simulink model "ModeAdjust"  (R2018b)
settings: Solver=FixedStepDiscrete  StartTime=0.0  StopTime=inf  FixedStep=0.01  RelTol=1e-3
undefined symbols (not defined in the file or in its folder): IfKeSMSbSeatMovBkRclnEnable_Val, IfKeSMSbSeatMovFrwdBkwdEnable_Val, IfKeSMSbSeatMovFtrstEnable_Val, IfKeSMSbSeatMovHdrstFrwdBkwdEnable_Val, IfKeSMSbSeatMovHdUpwdDnwdEnable_Val, IfKeSMSbSeatMovLgrstEnable_Val, IfKeSMSbSeatMovLtwdRtwdEnable_Val, IfVeSMSeStNumConfig, KeSMSbArmscreenMovEnable_Val, KeSMSbSeatMovLgrstExpdEnable_Val, KeSMSuFirstRwStBackPosDelta_Val, KeSMSuFirstRwStBackPosTolr_Val, KeSMSuFirstRwStCushFrntPosDelta_Val, KeSMSuFirstRwStCushFrntPosTolr_Val, KeSMSuFirstRwStCushRePosDelta_Val, KeSMSuFirstRwStCushRePosTolr_Val, KeSMSuFirstRwStFootrestPosDelta_Val, KeSMSuFirstRwStFootrestPosTolr_Val, KeSMSuFirstRwStFwdBkwdPosDelta_Val, KeSMSuFirstRwStFwdBkwdPosTolr_Val, KeSMSuMdMotFinshdTm_Val, KeSMSuMdRetryTm1_Val, KeSMSuModeReqDurgTm_Val, KeSMSuSecRwStArmTochPosDelta_Val, KeSMSuSecRwStArmTochPosTolr_Val, KeSMSuSecRwStBackPosDelta_Val, KeSMSuSecRwStBackPosTolr_Val, KeSMSuSecRwStFtrstUpwdDnwdPosDelta_Val, KeSMSuSecRwStFtrstUpwdDnwdPosTolr_Val, KeSMSuSecRwStFwdBkwdPosDelta_Val, KeSMSuSecRwStFwdBkwdPosTolr_Val, KeSMSuSecRwStHeadrestFwdBkwdPosDelta_Val, KeSMSuSecRwStHeadrestFwdBkwdPosTolr_Val, KeSMSuSecRwStHeadrestUpwdDwnwdPosDelta_Val, KeSMSuSecRwStHeadrestUpwdDwnwdPosTolr_Val, KeSMSuSecRwStLegrestInOutPosDelta_Val, KeSMSuSecRwStLegrestInOutPosTolr_Val, KeSMSuSecRwStLegrestUpwdDwnwdPosDelta_Val, KeSMSuSecRwStLegrestUpwdDwnwdPosTolr_Val, KeSMSuSecRwStLwdRwdPosDelta_Val, KeSMSuSecRwStLwdRwdPosTolr_Val, KeSMSuSecRwStVIPFtrstRefAngle_Val, KeSMSuThirdRwStFwdBkwdPosDelta_Val, KeSMSuThirdRwStFwdBkwdPosTolr_Val, KeSMSuThrdRwCushFoldPosDelta_Val, KeSMSuThrdRwCushFoldPosTolr_Val, KeSMSuThrdRwStBackPosDelta_Val, KeSMSuThrdRwStBackPosTolr_Val, KeSMSw4SLegrstCloseMdSecRwLtStFtrstUpwdDnwdPos_Val, KeSMSw4SLegrstCloseMdSecRwLtStFtrstUpwdDnwdPosMax_Val, KeSMSw4SLegrstCloseMdSecRwLtStFtrstUpwdDnwdPosMin_Val, KeSMSw4SLegrstCloseMdSecRwLtStLgrstOtwdInwdPos_Val, KeSMSw4SLegrstCloseMdSecRwLtStLgrstOtwdInwdPosMax_Val, KeSMSw4SLegrstCloseMdSecRwLtStLgrstOtwdInwdPosMin_Val, KeSMSw4SLegrstCloseMdSecRwLtStLgrstUpwdDnwdPos_Val, KeSMSw4SLegrstCloseMdSecRwLtStLgrstUpwdDnwdPosMax_Val, KeSMSw4SLegrstCloseMdSecRwLtStLgrstUpwdDnwdPosMin_Val, KeSMSw4SLegrstCloseMdSecRwRtStFtrstUpwdDnwdPos_Val, KeSMSw4SLegrstCloseMdSecRwRtStFtrstUpwdDnwdPosMax_Val, KeSMSw4SLegrstCloseMdSecRwRtStFtrstUpwdDnwdPosMin_Val ... (+1138)
libraries: Lib x401
(part 16 of 35)

== system ModeAdjust/ModeAdjustRunnable_sys/ModeAdjust/FAMLYR/R3Lt ==
  note: %1锁，2未锁
  Mode_Trig : Inport
  Step1En : Inport  Port=2
  ThdRwRtStPoss : Inport  Port=3
  ThdRwRtStPossV : Inport  Port=4
  ModeStCalib_3R : Inport  Port=5
  StConfig : Inport  Port=6
  SecRwRtStChldLkRsp_L : Inport  Port=7
  SecRwRtStChldLkRsp_R : Inport  Port=8
  Bus Creator : BusCreator  Inputs=3  OutDataTypeStr=Bus: ThdRwLfSeatPos
  Bus Selector : BusSelector  OutputSignals=IfVeSMSuThdRwLtStBkReclnUpwdDnwdPos_Val_read,IfVeSMSuThdRwLtStCshnFldUpwdDnwdPos_Val_read,IfVeSMSuThdRwLtStFrwdBkwdPos_Val_read
  Bus Selector1 : BusSelector  OutputSignals=IfVeSMSuThdRwLtStBkReclnUpwdDnwdPosV_Val_read,IfVeSMSuThdRwLtStCshnFldUpwdDnwdPosV_Val_read,IfVeSMSuThdRwLtStFrwdBkwdPosV_Val_read
  Bus Selector2 : BusSelector  OutputSignals=BkReclnUpwdDnwdPos,BkReclnUpwdDnwdPosMax,BkReclnUpwdDnwdPosMin,CshnFldUpwdDnwdPos,CshnFldUpwdDnwdPosMax,CshnFldUpwdDnwdPosMin,FrwdBkwdPos,FrwdBkwdPosMax,FrwdBkwdPosMin
  Bus Selector3 : BusSelector  OutputSignals=FamlyRThdRwLtSt
  Bus Selector4 : BusSelector  OutputSignals=BkReclnUpwdDnwdMovConfig,CshnFldUpwdDnwdMovConfig,FrwdBkwdMovConfig
  Constant : Constant  Value=2  OutDataTypeStr=uint8
  Constant1 : Constant  Value=0  OutDataTypeStr=uint8
  Logical Operator10 : Logic  Operator=OR  AllPortsSameDT=off  OutDataTypeStr=boolean
  Logical Operator6 : Logic  Operator=OR  AllPortsSameDT=off  OutDataTypeStr=boolean
  PA_KeSMSuMdMotFinshdTm_Val : Constant  Value=KeSMSuMdMotFinshdTm_Val
  PA_KeSMSuMdRetryTm1_Val : Constant  Value=KeSMSuMdRetryTm1_Val
  PA_KeSMSuModeReqDurgTm_Val : Constant  Value=KeSMSuModeReqDurgTm_Val
  PA_KeSMSuThirdRwStFwdBkwdPosDelta_Val : Constant  Value=KeSMSuThirdRwStFwdBkwdPosDelta_Val
  PA_KeSMSuThrdRwCushFoldPosDelta_Val : Constant  Value=KeSMSuThrdRwCushFoldPosDelta_Val
  PA_KeSMSuThrdRwStBackPosDelta_Val : Constant  Value=KeSMSuThrdRwStBackPosDelta_Val
  PA_KeSMSwDltTrgtPos_Val{1,6..7,18} (4 alike) : Constant  Value=KeSMSwPosInvalidVal_Val
  PA_KeSMSwDltTrgtPos_Val10 : Constant  OutDataTypeStr=boolean
  PA_KeSMSwDltTrgtPos_Val13 : Constant  Value=SeatChldLkSt.ChldLkSt_Unlock
  PA_KeSMSwDltTrgtPos_Val2 : Constant  Value=0  OutDataTypeStr=boolean
  PA_KeSMSwDltTrgtPos_Val3 : Constant  Value=0  OutDataTypeStr=boolean
  PA_KeSMSwDltTrgtPos_Val4 : Constant  Value=SeatChldLkSt.ChldLkSt_Unlock
  R3Rt_FrwdBkwd_Step2 : Lib/CommonUsed  SystemSampleTime=-1
  Relational Operator : RelationalOperator  Operator=~=  OutDataTypeStr=boolean  RndMeth=Simplest
  Relational Operator1 : RelationalOperator  Operator=~=  OutDataTypeStr=boolean  RndMeth=Simplest
  Relational Operator2 : RelationalOperator  Operator=~=  OutDataTypeStr=boolean  RndMeth=Simplest
  Switch : Switch  Criteria=u2 ~= 0
  Unit Delay : UnitDelay  SampleTime=-1
  R3Rt_Step1_ini : Outport
  R3Lt__Step1done : Outport  Port=2
  IfVeSMSbThdRwLtStRclCmdSrv_Val_writeRaw : Outport  Port=3
  R3Lt_TrgtPoss : Outport  Port=4  VectorParamsAs1DForOutWhenUnconnected=on
  R3Lt_SpdCtrl : Outport  Port=5  VectorParamsAs1DForOutWhenUnconnected=on
  wires:
  Bus Selector2/8 -> [K_FrwdBkwdPosMax]  "<FrwdBkwdPosMax>"
  Bus Selector2/1 -> [K_BkReclnUpwdDnwdPos]  "<BkReclnUpwdDnwdPos>"
  Bus Selector2/2 -> [K_BkReclnUpwdDnwdPosMax]  "<BkReclnUpwdDnwdPosMax>"
  Bus Selector2/9 -> [K_FrwdBkwdPosMin]  "<FrwdBkwdPosMin>"
  Bus Selector3/1 -> Bus Selector2/1  "<FamlyRThdRwLtSt>"
  Bus Selector2/3 -> [K_BkReclnUpwdDnwdPosMin]  "<BkReclnUpwdDnwdPosMin>"
  ModeStCalib_3R/1 -> Bus Selector3/1
  Bus Selector2/5 -> [K_CshnFldUpwdDnwdPosMax]  "<CshnFldUpwdDnwdPosMax>"
  Bus Selector2/7 -> [K_FrwdBkwdPos]  "<FrwdBkwdPos>"
  Bus Selector2/4 -> [K_CshnFldUpwdDnwdPos]  "<CshnFldUpwdDnwdPos>"
  Bus Selector2/6 -> [K_CshnFldUpwdDnwdPosMin]  "<CshnFldUpwdDnwdPosMin>"
  [KeSMSuMdMotFinshdTm_Val] -> R3Rt_FrwdBkwd_Step2/12
  PA_KeSMSuModeReqDurgTm_Val/1 -> [Tick]
  PA_KeSMSuMdMotFinshdTm_Val/1 -> [KeSMSuMdMotFinshdTm_Val]
  PA_KeSMSuThrdRwStBackPosDelta_Val/1 -> [KeSMSuThrdRwStBackPosDelta_Val]
  PA_KeSMSuThirdRwStFwdBkwdPosDelta_Val/1 -> [KeSMSuThirdRwStFwdBkwdPosDelta_Val]
  PA_KeSMSuThrdRwCushFoldPosDelta_Val/1 -> [KeSMSuThrdRwCushFoldPosDelta_Val]
  Logical Operator6/1 -> R3Lt__Step1done/1
  Unit Delay/1 -> Logical Operator6/2
  Step1En/1 -> R3Rt_FrwdBkwd_Step2/2
  [Step1_2_done] -> Unit Delay/1
  [R3Rt_Step1_2_ini] -> Logical Operator6/1, R3Rt_Step1_ini/1
  Mode_Trig/1 -> [Trig]
  [ThdRwRtStFrwdBkwdPos] -> R3Rt_FrwdBkwd_Step2/3
  [K_FrwdBkwdPosMax] -> R3Rt_FrwdBkwd_Step2/5
  [KeSMSuThirdRwStFwdBkwdPosDelta_Val] -> R3Rt_FrwdBkwd_Step2/7
  [K_FrwdBkwdPosMin] -> R3Rt_FrwdBkwd_Step2/4
  R3Rt_FrwdBkwd_Step2/1 -> [R3Rt_Step1_2_ini]
  R3Rt_FrwdBkwd_Step2/2 -> [Step2ArrivedTarPos]
  [Trig] -> R3Rt_FrwdBkwd_Step2/1
  [K_FrwdBkwdPos] -> R3Rt_FrwdBkwd_Step2/6
  [ThdRwRtStFrwdBkwdPosV] -> R3Rt_FrwdBkwd_Step2/8
  PA_KeSMSwDltTrgtPos_Val2/1 -> R3Rt_FrwdBkwd_Step2/9
  PA_KeSMSwDltTrgtPos_Val6/1 -> R3Rt_FrwdBkwd_Step2/10
  [Tick] -> R3Rt_FrwdBkwd_Step2/11
  R3Rt_FrwdBkwd_Step2/3 -> [R3Rt_FrwdBkwd_TarPos]
  R3Rt_FrwdBkwd_Step2/4 -> [Step1_2_done]
  Bus Selector1/1 -> [ThdRwRtStBkReclnUpwdDnwdPosV]  "<IfVeSMSuThdRwLtStBkReclnUpwdDnwdPosV_Val_read>"
  Bus Selector/3 -> [ThdRwRtStFrwdBkwdPos]  "<IfVeSMSuThdRwLtStFrwdBkwdPos_Val_read>"
  ThdRwRtStPossV/1 -> Bus Selector1/1
  ThdRwRtStPoss/1 -> Bus Selector/1
  Bus Selector/2 -> [ThdRwRtStCshnFldUpwdDnwdPos]  "<IfVeSMSuThdRwLtStCshnFldUpwdDnwdPos_Val_read>"
  Bus Selector/1 -> [ThdRwRtStBkReclnUpwdDnwdPos]  "<IfVeSMSuThdRwLtStBkReclnUpwdDnwdPos_Val_read>"
  Bus Selector1/2 -> [ThdRwRtStCshnFldUpwdDnwdPosV]  "<IfVeSMSuThdRwLtStCshnFldUpwdDnwdPosV_Val_read>"
  Bus Selector1/3 -> [ThdRwRtStFrwdBkwdPosV]  "<IfVeSMSuThdRwLtStFrwdBkwdPosV_Val_read>"
  PA_KeSMSwDltTrgtPos_Val1/1 -> Bus Creator/2  "ThdRwLtStCshnFldUpwdDnwdTrgtPos"
  PA_KeSMSwDltTrgtPos_Val7/1 -> Bus Creator/1  "ThdRwLtStBkReclnUpwdDnwdTrgtPos"
  [R3Rt_FrwdBkwd_TarPos] -> Bus Creator/3  "ThdRwLtStFrwdBkwdTrgtPos"
  Bus Creator/1 -> R3Lt_TrgtPoss/1
  Bus Selector4/1 -> [BkReclnUpwdDnwdMovConfig]  "<BkReclnUpwdDnwdMovConfig>"
  StConfig/1 -> Bus Selector4/1
  Bus Selector4/2 -> [CshnFldUpwdDnwdMovConfig]  "<CshnFldUpwdDnwdMovConfig>"
  Bus Selector4/3 -> [FrwdBkwdMovConfig]  "<FrwdBkwdMovConfig>"
  [FrwdBkwdMovConfig] -> R3Rt_FrwdBkwd_Step2/14
  PA_KeSMSwDltTrgtPos_Val10/1 -> IfVeSMSbThdRwLtStRclCmdSrv_Val_writeRaw/1
  PA_KeSMSwDltTrgtPos_Val3/1 -> R3Rt_FrwdBkwd_Step2/13
  PA_KeSMSwDltTrgtPos_Val13/1 -> Relational Operator1/2
  SecRwRtStChldLkRsp_R/1 -> Relational Operator1/1
  Relational Operator1/1 -> Logical Operator10/2
  SecRwRtStChldLkRsp_L/1 -> Relational Operator/1
  Relational Operator/1 -> Logical Operator10/1
  Logical Operator10/1 -> [ChildLocker]
  PA_KeSMSwDltTrgtPos_Val4/1 -> Relational Operator/2
  [CntLow] -> R3Rt_FrwdBkwd_Step2/15
  PA_KeSMSuMdRetryTm1_Val/1 -> [CntLow]
  [R3Rt_FrwdBkwd_TarPos] -> Relational Operator2/1  "ThdRwLtStFrwdBkwdTrgtPos"
  PA_KeSMSwDltTrgtPos_Val18/1 -> Relational Operator2/2
  Switch/1 -> R3Lt_SpdCtrl/1
  Relational Operator2/1 -> Switch/2
  Constant1/1 -> Switch/3
  Constant/1 -> Switch/1

== system ModeAdjust/ModeAdjustRunnable_sys/ModeAdjust/FAMLYR/R3Rt ==
  note: %1锁，2未锁
  Mode_Trig : Inport
  Step1En : Inport  Port=2
  ThdRwRtStPoss : Inport  Port=3
  ThdRwRtStPossV : Inport  Port=4
  ModeStCalib_3R : Inport  Port=5
  StConfig : Inport  Port=6
  SecRwRtStChldLkRsp_L : Inport  Port=7
  SecRwRtStChldLkRsp_R : Inport  Port=8
  Bus Creator : BusCreator  Inputs=3  OutDataTypeStr=Bus: ThdRwRtSeatPos
  Bus Selector : BusSelector  OutputSignals=IfVeSMSuThdRwRtStBkReclnUpwdDnwdPos_Val_read,IfVeSMSuThdRwRtStCshnFldUpwdDnwdPos_Val_read,IfVeSMSuThdRwRtStFrwdBkwdPos_Val_read
  Bus Selector1 : BusSelector  OutputSignals=IfVeSMSuThdRwRtStBkReclnUpwdDnwdPosV_Val_read,IfVeSMSuThdRwRtStCshnFldUpwdDnwdPosV_Val_read,IfVeSMSuThdRwRtStFrwdBkwdPosV_Val_read
  Bus Selector2 : BusSelector  OutputSignals=BkReclnUpwdDnwdPos,BkReclnUpwdDnwdPosMax,BkReclnUpwdDnwdPosMin,CshnFldUpwdDnwdPos,CshnFldUpwdDnwdPosMax,CshnFldUpwdDnwdPosMin,FrwdBkwdPos,FrwdBkwdPosMax,FrwdBkwdPosMin
  Bus Selector3 : BusSelector  OutputSignals=FamlyRThdRwRtSt
  Bus Selector4 : BusSelector  OutputSignals=BkReclnUpwdDnwdMovConfig,CshnFldUpwdDnwdMovConfig,FrwdBkwdMovConfig
  Constant : Constant  Value=2  OutDataTypeStr=uint8
  Constant1 : Constant  Value=0  OutDataTypeStr=uint8
  Logical Operator6 : Logic  Operator=OR  AllPortsSameDT=off  OutDataTypeStr=boolean
  Logical Operator9 : Logic  Operator=OR  AllPortsSameDT=off  OutDataTypeStr=boolean
  PA_KeSMSuMdMotFinshdTm_Val : Constant  Value=KeSMSuMdMotFinshdTm_Val
  PA_KeSMSuMdRetryTm1_Val : Constant  Value=KeSMSuMdRetryTm1_Val
  PA_KeSMSuModeReqDurgTm_Val : Constant  Value=KeSMSuModeReqDurgTm_Val
  PA_KeSMSuThirdRwStFwdBkwdPosDelta_Val : Constant  Value=KeSMSuThirdRwStFwdBkwdPosDelta_Val
  PA_KeSMSuThrdRwCushFoldPosDelta_Val : Constant  Value=KeSMSuThrdRwCushFoldPosDelta_Val
  PA_KeSMSuThrdRwStBackPosDelta_Val : Constant  Value=KeSMSuThrdRwStBackPosDelta_Val
  PA_KeSMSwDltTrgtPos_Val{1,6..7,18} (4 alike) : Constant  Value=KeSMSwPosInvalidVal_Val
  PA_KeSMSwDltTrgtPos_Val10 : Constant  OutDataTypeStr=boolean
  PA_KeSMSwDltTrgtPos_Val12 : Constant  Value=SeatChldLkSt.ChldLkSt_Unlock
  PA_KeSMSwDltTrgtPos_Val2 : Constant  Value=0  OutDataTypeStr=boolean
  PA_KeSMSwDltTrgtPos_Val3 : Constant  Value=0  OutDataTypeStr=boolean
  PA_KeSMSwDltTrgtPos_Val9 : Constant  Value=SeatChldLkSt.ChldLkSt_Unlock
  R3Rt_FrwdBkwd_Step2 : Lib/CommonUsed  SystemSampleTime=-1
  Relational Operator1 : RelationalOperator  Operator=~=  OutDataTypeStr=boolean  RndMeth=Simplest
  Relational Operator2 : RelationalOperator  Operator=~=  OutDataTypeStr=boolean  RndMeth=Simplest
  Relational Operator3 : RelationalOperator  Operator=~=  OutDataTypeStr=boolean  RndMeth=Simplest
  Switch : Switch  Criteria=u2 ~= 0
  Unit Delay : UnitDelay  SampleTime=-1
  R3Rt_Step1_ini : Outport
  R3Rt__Step1done : Outport  Port=2
  IfVeSMSbThdRwRtStRclCmdSrv_Val_writeRaw : Outport  Port=3
  R3Rt_TrgtPoss : Outport  Port=4  VectorParamsAs1DForOutWhenUnconnected=on
  R3Rt_SpdCtrl : Outport  Port=5  VectorParamsAs1DForOutWhenUnconnected=on
  wires:
  Bus Selector2/8 -> [K_FrwdBkwdPosMax]  "<FrwdBkwdPosMax>"
  Bus Selector2/1 -> [K_BkReclnUpwdDnwdPos]  "<BkReclnUpwdDnwdPos>"
  Bus Selector2/2 -> [K_BkReclnUpwdDnwdPosMax]  "<BkReclnUpwdDnwdPosMax>"
  Bus Selector2/9 -> [K_FrwdBkwdPosMin]  "<FrwdBkwdPosMin>"
  Bus Selector3/1 -> Bus Selector2/1  "<FamlyRThdRwRtSt>"
  Bus Selector2/3 -> [K_BkReclnUpwdDnwdPosMin]  "<BkReclnUpwdDnwdPosMin>"
  ModeStCalib_3R/1 -> Bus Selector3/1
  Bus Selector2/5 -> [K_CshnFldUpwdDnwdPosMax]  "<CshnFldUpwdDnwdPosMax>"
  Bus Selector2/7 -> [K_FrwdBkwdPos]  "<FrwdBkwdPos>"
  Bus Selector2/4 -> [K_CshnFldUpwdDnwdPos]  "<CshnFldUpwdDnwdPos>"
  Bus Selector2/6 -> [K_CshnFldUpwdDnwdPosMin]  "<CshnFldUpwdDnwdPosMin>"
  [KeSMSuMdMotFinshdTm_Val] -> R3Rt_FrwdBkwd_Step2/12
  PA_KeSMSuModeReqDurgTm_Val/1 -> [Tick]
  PA_KeSMSuMdMotFinshdTm_Val/1 -> [KeSMSuMdMotFinshdTm_Val]
  PA_KeSMSuThrdRwStBackPosDelta_Val/1 -> [KeSMSuThrdRwStBackPosDelta_Val]
  PA_KeSMSuThirdRwStFwdBkwdPosDelta_Val/1 -> [KeSMSuThirdRwStFwdBkwdPosDelta_Val]
  PA_KeSMSuThrdRwCushFoldPosDelta_Val/1 -> [KeSMSuThrdRwCushFoldPosDelta_Val]
  Logical Operator6/1 -> R3Rt__Step1done/1
  Unit Delay/1 -> Logical Operator6/2
  Step1En/1 -> R3Rt_FrwdBkwd_Step2/2
  [Step1_2_done] -> Unit Delay/1
  [R3Rt_Step1_2_ini] -> Logical Operator6/1, R3Rt_Step1_ini/1
  Mode_Trig/1 -> [Trig]
  [ThdRwRtStFrwdBkwdPos] -> R3Rt_FrwdBkwd_Step2/3
  [K_FrwdBkwdPosMax] -> R3Rt_FrwdBkwd_Step2/5
  [KeSMSuThirdRwStFwdBkwdPosDelta_Val] -> R3Rt_FrwdBkwd_Step2/7
  [K_FrwdBkwdPosMin] -> R3Rt_FrwdBkwd_Step2/4
  R3Rt_FrwdBkwd_Step2/1 -> [R3Rt_Step1_2_ini]
  R3Rt_FrwdBkwd_Step2/2 -> [Step2ArrivedTarPos]
  [Trig] -> R3Rt_FrwdBkwd_Step2/1
  [K_FrwdBkwdPos] -> R3Rt_FrwdBkwd_Step2/6
  [ThdRwRtStFrwdBkwdPosV] -> R3Rt_FrwdBkwd_Step2/8
  PA_KeSMSwDltTrgtPos_Val2/1 -> R3Rt_FrwdBkwd_Step2/9
  PA_KeSMSwDltTrgtPos_Val6/1 -> R3Rt_FrwdBkwd_Step2/10
  [Tick] -> R3Rt_FrwdBkwd_Step2/11
  R3Rt_FrwdBkwd_Step2/3 -> [R3Rt_FrwdBkwd_TarPos]
  R3Rt_FrwdBkwd_Step2/4 -> [Step1_2_done]
  Bus Selector1/1 -> [ThdRwRtStBkReclnUpwdDnwdPosV]  "<IfVeSMSuThdRwRtStBkReclnUpwdDnwdPosV_Val_read>"
  Bus Selector/3 -> [ThdRwRtStFrwdBkwdPos]  "<IfVeSMSuThdRwRtStFrwdBkwdPos_Val_read>"
  ThdRwRtStPossV/1 -> Bus Selector1/1
  ThdRwRtStPoss/1 -> Bus Selector/1
  Bus Selector/2 -> [ThdRwRtStCshnFldUpwdDnwdPos]  "<IfVeSMSuThdRwRtStCshnFldUpwdDnwdPos_Val_read>"
  Bus Selector/1 -> [ThdRwRtStBkReclnUpwdDnwdPos]  "<IfVeSMSuThdRwRtStBkReclnUpwdDnwdPos_Val_read>"
  Bus Selector1/2 -> [ThdRwRtStCshnFldUpwdDnwdPosV]  "<IfVeSMSuThdRwRtStCshnFldUpwdDnwdPosV_Val_read>"
  Bus Selector1/3 -> [ThdRwRtStFrwdBkwdPosV]  "<IfVeSMSuThdRwRtStFrwdBkwdPosV_Val_read>"
  PA_KeSMSwDltTrgtPos_Val1/1 -> Bus Creator/2  "ThdRwRtStCshnFldUpwdDnwdTrgtPos"
  PA_KeSMSwDltTrgtPos_Val7/1 -> Bus Creator/1  "ThdRwRtStBkReclnUpwdDnwdTrgtPos"
  [R3Rt_FrwdBkwd_TarPos] -> Bus Creator/3  "ThdRwRtStFrwdBkwdTrgtPos"
  Bus Creator/1 -> R3Rt_TrgtPoss/1
  Bus Selector4/1 -> [BkReclnUpwdDnwdMovConfig]  "<BkReclnUpwdDnwdMovConfig>"
  StConfig/1 -> Bus Selector4/1
  Bus Selector4/2 -> [CshnFldUpwdDnwdMovConfig]  "<CshnFldUpwdDnwdMovConfig>"
  Bus Selector4/3 -> [FrwdBkwdMovConfig]  "<FrwdBkwdMovConfig>"
  [FrwdBkwdMovConfig] -> R3Rt_FrwdBkwd_Step2/14
  PA_KeSMSwDltTrgtPos_Val9/1 -> Relational Operator1/2
  SecRwRtStChldLkRsp_L/1 -> Relational Operator1/1
  Logical Operator9/1 -> [ChildLocker]
  PA_KeSMSwDltTrgtPos_Val10/1 -> IfVeSMSbThdRwRtStRclCmdSrv_Val_writeRaw/1
  PA_KeSMSwDltTrgtPos_Val3/1 -> R3Rt_FrwdBkwd_Step2/13
  Relational Operator1/1 -> Logical Operator9/1
  Relational Operator2/1 -> Logical Operator9/2
  SecRwRtStChldLkRsp_R/1 -> Relational Operator2/1
  PA_KeSMSwDltTrgtPos_Val12/1 -> Relational Operator2/2
  [CntLow] -> R3Rt_FrwdBkwd_Step2/15
  PA_KeSMSuMdRetryTm1_Val/1 -> [CntLow]
  Relational Operator3/1 -> Switch/2
  PA_KeSMSwDltTrgtPos_Val18/1 -> Relational Operator3/2
  Switch/1 -> R3Rt_SpdCtrl/1
  [R3Rt_FrwdBkwd_TarPos] -> Relational Operator3/1
  Constant1/1 -> Switch/3
  Constant/1 -> Switch/1

== system ModeAdjust/ModeAdjustRunnable_sys/ModeAdjust/INTML/R2Lt ==
  note: %1锁，2未锁
  Mode_Trig : Inport
  Step1En : Inport  Port=2
  SecRwLtStsPoss : Inport  Port=3
  SecRwLtStPossV : Inport  Port=4
  SecRwRtStChldLkRsp_L : Inport  Port=5
  ModeStCalib_2L : Inport  Port=6
  StConfig : Inport  Port=7
  SecRwRtStChldLkRsp_R : Inport  Port=8
  SecRwRtStPoss : Inport  Port=9
  Bus Creator : BusCreator  Inputs=9  OutDataTypeStr=Bus: SecRwLfSeatPos
  Bus Selector : BusSelector  OutputSignals=IfVeSMSuSecRwLtStBkReclnUpwdDnwdPos_Val_read,IfVeSMSuSecRwLtStFrwdBkwdPos_Val_read,IfVeSMSuSecRwLtStHPassStUpwdDnwdPos_Val_read,IfVeSMSuSecRwLtStLgrstUpwdDnwdPos_Val_read,IfVeSMSuSecRwLtStLtwdRtwdPos_Val_read,IfVeSMSuSecRwLtStArmScrnPos_Val_read
  Bus Selector1 : BusSelector  OutputSignals=IfVeSMSuSecRwLtStBkReclnUpwdDnwdPosV_Val_read,IfVeSMSuSecRwLtStFrwdBkwdPosV_Val_read,IfVeSMSuSecRwLtStHPassStUpwdDnwdPosV_Val_read,IfVeSMSuSecRwLtStLgrstUpwdDnwdPosV_Val_read,IfVeSMSuSecRwLtStLtwdRtwdPosV_Val_read,IfVeSMSuSecRwLtStArmScrnPosV_Val_read
  Bus Selector2 : BusSelector  OutputSignals=ArmScrnPos,ArmScrnPosMax,ArmScrnPosMin,BkReclnUpwdDnwdPos,BkReclnUpwdDnwdPosMax,BkReclnUpwdDnwdPosMin,FrwdBkwdPos,FrwdBkwdPosMax,FrwdBkwdPosMin,HdrstUpwdPos,HdrstUpwdPosMax,HdrstUpwdPosMin,LgrstUpwdPos,LgrstUpwdPosMax,LgrstUpwdPosMin,LtwdRtwdPos,LtwdRtwdPosMax,LtwdRtwdPosMin
  Bus Selector3 : BusSelector  OutputSignals=INTMSecRwLtSt
  Bus Selector4 : BusSelector  OutputSignals=BkReclnUpwdDnwdMovConfig,ArmTouchMovConfig,FrwdBkwdMovConfig,LgrstUpwdMovConfig,LtwdRtwdMovConfig
  Bus Selector5 : BusSelector  OutputSignals=IfVeSMSuSecRwRtStBkReclnUpwdDnwdPos_Val_read,IfVeSMSuSecRwRtStFrwdBkwdPos_Val_read,IfVeSMSuSecRwRtStHPassStUpwdDnwdPos_Val_read,IfVeSMSuSecRwRtStLgrstUpwdDnwdPos_Val_read,IfVeSMSuSecRwRtStLtwdRtwdPos_Val_read,SecRwRtStArmScrnPos_Val_read
  Constant : Constant  Value=2  OutDataTypeStr=uint8
  Constant1 : Constant  Value=0  OutDataTypeStr=uint8
  Logical Operator1 : Logic  AllPortsSameDT=off  OutDataTypeStr=boolean
  Logical Operator3 : Logic  Operator=OR  AllPortsSameDT=off  OutDataTypeStr=boolean
  Logical Operator4 : Logic  AllPortsSameDT=off  OutDataTypeStr=boolean
  PA_KeSMSuMdMotFinshdTm_Val : Constant  Value=KeSMSuMdMotFinshdTm_Val
  PA_KeSMSuMdRetryTm1_Val : Constant  Value=KeSMSuMdRetryTm1_Val
  PA_KeSMSuModeReqDurgTm_Val : Constant  Value=KeSMSuModeReqDurgTm_Val
  PA_KeSMSuSecRwStArmTochPosDelta_Val : Constant  Value=KeSMSuSecRwStArmTochPosDelta_Val
  PA_KeSMSuSecRwStBackPosDelta_Val : Constant  Value=KeSMSuSecRwStBackPosDelta_Val
  PA_KeSMSuSecRwStFwdBkwdPosDelta_Val : Constant  Value=KeSMSuSecRwStFwdBkwdPosDelta_Val
  PA_KeSMSuSecRwStLegrestUpwdDwnwdPosDelta_Val : Constant  Value=KeSMSuSecRwStLegrestUpwdDwnwdPosDelta_Val
  PA_KeSMSuSecRwStLwdRwdPosDelta_Val : Constant  Value=KeSMSuSecRwStLwdRwdPosDelta_Val
  PA_KeSMSwDltTrgtPos_Val{1,3..4,6,11,14,18..21} (10 alike) : Constant  Value=KeSMSwPosInvalidVal_Val
  PA_KeSMSwDltTrgtPos_Val{8..10,12} (4 alike) : Constant  Value=0  OutDataTypeStr=boolean
  PA_KeSMSwDltTrgtPos_Val2 : Constant  Value=SeatChldLkSt.ChldLkSt_Unlock
  PA_KeSMSwDltTrgtPos_Val5 : Constant  OutDataTypeStr=boolean
  PA_KeSMSwDltTrgtPos_Val7 : Constant  Value=SeatChldLkSt.ChldLkSt_Unlock
  R2LtSt_FrwdBkwd : Lib/CommonUsed  SystemSampleTime=-1
  R2LtSt_LtwdRtwd_Step3 : Lib/CommonUsed  SystemSampleTime=-1
  Relational Operator1 : RelationalOperator  Operator=~=  OutDataTypeStr=boolean  RndMeth=Simplest
  Switch : Switch  Criteria=u2 ~= 0
  Terminator{,1..5} (6 alike) : Terminator
  Unit Delay : UnitDelay  SampleTime=-1
  Unit Delay1 : UnitDelay  SampleTime=-1
  R2Lt_Ini : Outport
  R2Lt_Step2_done : Outport  Port=2
  R2Lt_TrgtPoss : Outport  Port=3  VectorParamsAs1DForOutWhenUnconnected=on
  IfVeSMSuSecRwLtStRclCmdSrv_Val_writeRaw : Outport  Port=4
  R2Lt_SpdCtrl : Outport  Port=5  VectorParamsAs1DForOutWhenUnconnected=on
  wires:
  PA_KeSMSwDltTrgtPos_Val20/1 -> Bus Creator/4  "SecRwLtStCshnRrUpwdDnwdTrgtPos"
  [R2LtStFrwdBkwd_TarPos] -> Bus Creator/5  "SecRwLtStFrwdBkwdTrgtPos"
  PA_KeSMSwDltTrgtPos_Val1/1 -> Bus Creator/1  "SecRwLtStBkReclnUpwdDnwdTrgtPos"
  PA_KeSMSwDltTrgtPos_Val18/1 -> Bus Creator/2  "SecRwLtStBlstOtwdInwdTrgtPos"
  [R2LtSt_LtwdRtwd_TarPos] -> Bus Creator/8  "SecRwLtStLtwdRtwdTrgtPos"
  PA_KeSMSwDltTrgtPos_Val19/1 -> Bus Creator/3  "SecRwLtStCshnFrntUpwdDnwdTrgtPos"
  PA_KeSMSwDltTrgtPos_Val4/1 -> Bus Creator/7  "SecRwLtStLgrstUpwdDnwdTrgtPos"
  Bus Creator/1 -> R2Lt_TrgtPoss/1
  PA_KeSMSwDltTrgtPos_Val21/1 -> Bus Creator/6  "SecRwLtStHdrstUpwdDnwdTrgtPos"
  R2LtSt_LtwdRtwd_Step3/2 -> Terminator4/1
  [LtwdRtwd_done] -> Unit Delay/1
  [Step1En] -> R2LtSt_LtwdRtwd_Step3/2
  R2LtSt_LtwdRtwd_Step3/3 -> [R2LtSt_LtwdRtwd_TarPos]
  R2LtSt_LtwdRtwd_Step3/1 -> [LtwdRtwd_inidone]
  R2LtSt_LtwdRtwd_Step3/4 -> [LtwdRtwd_done]
  PA_KeSMSwDltTrgtPos_Val8/1 -> R2LtSt_LtwdRtwd_Step3/9
  [KeSMSuSecRwStLwdRwdPosDelta_Val] -> R2LtSt_LtwdRtwd_Step3/7
  [Tick] -> R2LtSt_LtwdRtwd_Step3/11
  PA_KeSMSwDltTrgtPos_Val14/1 -> R2LtSt_LtwdRtwd_Step3/10
  [Trig] -> R2LtSt_LtwdRtwd_Step3/1
  [SecRwLtStLtwdRtwdPosV] -> R2LtSt_LtwdRtwd_Step3/8
  [SecRwLtStLtwdRtwdPos] -> R2LtSt_LtwdRtwd_Step3/3
  [K_LtwdRtwdPosMin] -> R2LtSt_LtwdRtwd_Step3/4
  [K_LtwdRtwdPos] -> R2LtSt_LtwdRtwd_Step3/6
  [K_LtwdRtwdPosMax] -> R2LtSt_LtwdRtwd_Step3/5
  PA_KeSMSwDltTrgtPos_Val2/1 -> Terminator1/1
  SecRwRtStChldLkRsp_L/1 -> Terminator/1
  Bus Selector/1 -> [SecRwLtStBkReclnUpwdDnwdPos]  "<IfVeSMSuSecRwLtStBkReclnUpwdDnwdPos_Val_read>"
  Bus Selector1/2 -> [SecRwLtStFrwdBkwdPosV]  "<IfVeSMSuSecRwLtStFrwdBkwdPosV_Val_read>"
  Bus Selector1/1 -> [SecRwLtStBkReclnUpwdDnwdPosV]  "<IfVeSMSuSecRwLtStBkReclnUpwdDnwdPosV_Val_read>"
  Bus Selector/2 -> [SecRwLtStFrwdBkwdPos]  "<IfVeSMSuSecRwLtStFrwdBkwdPos_Val_read>"
  Bus Selector/4 -> [SecRwLtStLgrstUpwdDnwdPos]  "<IfVeSMSuSecRwLtStLgrstUpwdDnwdPos_Val_read>"
  Bus Selector1/5 -> [SecRwLtStLtwdRtwdPosV]  "<IfVeSMSuSecRwLtStLtwdRtwdPosV_Val_read>"
  Bus Selector/3 -> [SecRwLtStHPassStUpwdDnwdPos]  "<IfVeSMSuSecRwLtStHPassStUpwdDnwdPos_Val_read>"
  SecRwLtStPossV/1 -> Bus Selector1/1
  Bus Selector1/4 -> [SecRwLtStLgrstUpwdDnwdPosV]  "<IfVeSMSuSecRwLtStLgrstUpwdDnwdPosV_Val_read>"
  SecRwLtStsPoss/1 -> Bus Selector/1
  Bus Selector/5 -> [SecRwLtStLtwdRtwdPos]  "<IfVeSMSuSecRwLtStLtwdRtwdPos_Val_read>"
  Bus Selector1/3 -> [SecRwLtStHPassStUpwdDnwdPosV]  "<IfVeSMSuSecRwLtStHPassStUpwdDnwdPosV_Val_read>"
  Mode_Trig/1 -> [Trig]
  Step1En/1 -> [Step1En]
  PA_KeSMSwDltTrgtPos_Val5/1 -> IfVeSMSuSecRwLtStRclCmdSrv_Val_writeRaw/1
  PA_KeSMSuModeReqDurgTm_Val/1 -> [Tick]
  PA_KeSMSwDltTrgtPos_Val6/1 -> Bus Creator/9  "SecRwLtStArmScrnTrgtPos"
  PA_KeSMSuSecRwStBackPosDelta_Val/1 -> [KeSMSuSecRwStBackPosDelta_Val]
  PA_KeSMSuMdMotFinshdTm_Val/1 -> [KeSMSuMdMotFinshdTm_Val]
  PA_KeSMSuSecRwStFwdBkwdPosDelta_Val/1 -> [KeSMSuSecRwStFwdBkwdPosDelta_Val]
  PA_KeSMSuSecRwStLwdRwdPosDelta_Val/1 -> [KeSMSuSecRwStLwdRwdPosDelta_Val]
  PA_KeSMSuSecRwStArmTochPosDelta_Val/1 -> [KeSMSuSecRwStArmTochPosDelta_Val]
  PA_KeSMSuSecRwStLegrestUpwdDwnwdPosDelta_Val/1 -> [KeSMSuSecRwStLegrestUpwdDwnwdPosDelta_Val]
  [KeSMSuMdMotFinshdTm_Val] -> R2LtSt_LtwdRtwd_Step3/12
  Bus Selector/6 -> [SecRwLtStArmScrnPos]  "<IfVeSMSuSecRwLtStArmScrnPos_Val_read>"
  Bus Selector1/6 -> [SecRwLtStArmScrnPosV]  "<IfVeSMSuSecRwLtStArmScrnPosV_Val_read>"
  Bus Selector2/1 -> [K_ArmScrnPos]  "<ArmScrnPos>"
  Bus Selector2/18 -> [K_LtwdRtwdPosMin]  "<LtwdRtwdPosMin>"
  Bus Selector2/16 -> [K_LtwdRtwdPos]  "<LtwdRtwdPos>"
  Bus Selector2/15 -> [K_LgrstUpwdPosMin]  "<LgrstUpwdPosMin>"
  Bus Selector2/17 -> [K_LtwdRtwdPosMax]  "<LtwdRtwdPosMax>"
  Bus Selector2/12 -> [K_HdrstUpwdPosMin]  "<HdrstUpwdPosMin>"
  Bus Selector2/13 -> [K_LgrstUpwdPos]  "<LgrstUpwdPos>"
  Bus Selector2/11 -> [K_HdrstUpwdPosMax]  "<HdrstUpwdPosMax>"
  Bus Selector2/14 -> [K_LgrstUpwdPosMax]  "<LgrstUpwdPosMax>"
  Bus Selector2/10 -> [K_HdrstUpwdPos]  "<HdrstUpwdPos>"
  Bus Selector2/4 -> [K_BkReclnUpwdDnwdPos]  "<BkReclnUpwdDnwdPos>"
  Bus Selector2/9 -> [K_FrwdBkwdPosMin]  "<FrwdBkwdPosMin>"
  Bus Selector2/5 -> [K_BkReclnUpwdDnwdPosMax]  "<BkReclnUpwdDnwdPosMax>"
  Bus Selector2/8 -> [K_FrwdBkwdPosMax]  "<FrwdBkwdPosMax>"
  Bus Selector3/1 -> Bus Selector2/1  "<INTMSecRwLtSt>"
  Bus Selector2/7 -> [K_FrwdBkwdPos]  "<FrwdBkwdPos>"
  Bus Selector2/3 -> [K_ArmScrnPosMin]  "<ArmScrnPosMin>"
  Bus Selector2/2 -> [K_ArmScrnPosMax]  "<ArmScrnPosMax>"
  Bus Selector2/6 -> [K_BkReclnUpwdDnwdPosMin]  "<BkReclnUpwdDnwdPosMin>"
  ModeStCalib_2L/1 -> Bus Selector3/1
  PA_KeSMSwDltTrgtPos_Val9/1 -> R2LtSt_LtwdRtwd_Step3/13
  StConfig/1 -> Bus Selector4/1
  Bus Selector4/4 -> [LgrstUpwdMovConfig]  "<LgrstUpwdMovConfig>"
  Bus Selector4/3 -> [FrwdBkwdMovConfig]  "<FrwdBkwdMovConfig>"
  Bus Selector4/2 -> [ArmTouchMovConfig]  "<ArmTouchMovConfig>"
  Bus Selector4/1 -> [BkReclnUpwdDnwdMovConfig]  "<BkReclnUpwdDnwdMovConfig>"
  Bus Selector4/5 -> [LtwdRtwdMovConfig]  "<LtwdRtwdMovConfig>"
  [LtwdRtwdMovConfig] -> R2LtSt_LtwdRtwd_Step3/14
  SecRwRtStChldLkRsp_R/1 -> Terminator2/1
  PA_KeSMSwDltTrgtPos_Val7/1 -> Terminator3/1
  [CntLow] -> R2LtSt_LtwdRtwd_Step3/15
  PA_KeSMSuMdRetryTm1_Val/1 -> [CntLow]
  [KeSMSuSecRwStFwdBkwdPosDelta_Val] -> R2LtSt_FrwdBkwd/7
  [KeSMSuMdMotFinshdTm_Val] -> R2LtSt_FrwdBkwd/12
  [SecRwRtStFrwdBkwdPos] -> R2LtSt_FrwdBkwd/5
  R2LtSt_FrwdBkwd/3 -> [R2LtStFrwdBkwd_TarPos]
  [SecRwLtStFrwdBkwdPosV] -> R2LtSt_FrwdBkwd/8
  R2LtSt_FrwdBkwd/1 -> [R2Lt_FrwdBkwd_ini]
  [Trig] -> R2LtSt_FrwdBkwd/1
  [Tick] -> R2LtSt_FrwdBkwd/11
  PA_KeSMSwDltTrgtPos_Val12/1 -> R2LtSt_FrwdBkwd/9
  [Step1En] -> R2LtSt_FrwdBkwd/2
  R2LtSt_FrwdBkwd/2 -> Terminator5/1
  [SecRwRtStFrwdBkwdPos] -> R2LtSt_FrwdBkwd/4
  [CntLow] -> R2LtSt_FrwdBkwd/15
  [FrwdBkwdMovConfig] -> R2LtSt_FrwdBkwd/14
  PA_KeSMSwDltTrgtPos_Val3/1 -> R2LtSt_FrwdBkwd/10
  [SecRwLtStFrwdBkwdPos] -> R2LtSt_FrwdBkwd/3
  PA_KeSMSwDltTrgtPos_Val10/1 -> R2LtSt_FrwdBkwd/13
  [SecRwRtStFrwdBkwdPos] -> R2LtSt_FrwdBkwd/6
  R2LtSt_FrwdBkwd/4 -> [FrwdBkwd_done]
  Unit Delay1/1 -> Logical Operator1/2
  [FrwdBkwd_done] -> Unit Delay1/1
  Unit Delay/1 -> Logical Operator1/1
  Logical Operator4/1 -> Logical Operator3/1, R2Lt_Ini/1
  Logical Operator1/1 -> Logical Operator3/2
  Logical Operator3/1 -> R2Lt_Step2_done/1
  [LtwdRtwd_inidone] -> Logical Operator4/1
  [R2Lt_FrwdBkwd_ini] -> Logical Operator4/2
  Bus Selector5/3 -> [SecRwRtStHPassStUpwdDnwdPos]  "<IfVeSMSuSecRwRtStHPassStUpwdDnwdPos_Val_read>"
  Bus Selector5/2 -> [SecRwRtStFrwdBkwdPos]  "<IfVeSMSuSecRwRtStFrwdBkwdPos_Val_read>"
  Bus Selector5/5 -> [SecRwRtStLtwdRtwdPos]  "<IfVeSMSuSecRwRtStLtwdRtwdPos_Val_read>"
  Bus Selector5/1 -> [SecRwRtStBkReclnUpwdDnwdPos]  "<IfVeSMSuSecRwRtStBkReclnUpwdDnwdPos_Val_read>"
  SecRwRtStPoss/1 -> Bus Selector5/1
  Bus Selector5/4 -> [SecRwRtStLgrstUpwdDnwdPos]  "<IfVeSMSuSecRwRtStLgrstUpwdDnwdPos_Val_read>"
  Bus Selector5/6 -> [SecRwRtStArmScrnPos]  "<SecRwRtStArmScrnPos_Val_read>"
  Switch/1 -> R2Lt_SpdCtrl/1
  [R2LtStFrwdBkwd_TarPos] -> Relational Operator1/1
  Relational Operator1/1 -> Switch/2
  Constant1/1 -> Switch/3
  Constant/1 -> Switch/1
  PA_KeSMSwDltTrgtPos_Val11/1 -> Relational Operator1/2

== system ModeAdjust/ModeAdjustRunnable_sys/ModeAdjust/INTML/R2Rt ==
  note: %1锁，2未锁
  Mode_Trig : Inport
  Step1En : Inport  Port=2
  SecRwRtStPoss : Inport  Port=3
  SecRwRtStPossV : Inport  Port=4
  SecRwRtStChldLkRsp_L : Inport  Port=5
  ModeStCalib_2R : Inport  Port=6
  StConfig : Inport  Port=7
  SecRwRtStChldLkRsp_R : Inport  Port=8
  Bus Creator : BusCreator  Inputs=9  OutDataTypeStr=Bus: SecRwRtSeatPos
  Bus Selector : BusSelector  OutputSignals=IfVeSMSuSecRwRtStBkReclnUpwdDnwdPos_Val_read,IfVeSMSuSecRwRtStFrwdBkwdPos_Val_read,IfVeSMSuSecRwRtStHPassStUpwdDnwdPos_Val_read,IfVeSMSuSecRwRtStLgrstUpwdDnwdPos_Val_read,IfVeSMSuSecRwRtStLtwdRtwdPos_Val_read,SecRwRtStArmScrnPos_Val_read
  Bus Selector1 : BusSelector  OutputSignals=IfVeSMSuSecRwRtStBkReclnUpwdDnwdPosV_Val_read,IfVeSMSuSecRwRtStFrwdBkwdPosV_Val_read,IfVeSMSuSecRwRtStHPassStUpwdDnwdPosV_Val_read,IfVeSMSuSecRwRtStLgrstUpwdDnwdPosV_Val_read,IfVeSMSuSecRwRtStLtwdRtwdPosV_Val_read,SecRwRtStArmScrnPosV_Val_read
  Bus Selector2 : BusSelector  OutputSignals=ArmScrnPos,ArmScrnPosMax,ArmScrnPosMin,BkReclnUpwdDnwdPos,BkReclnUpwdDnwdPosMax,BkReclnUpwdDnwdPosMin,FrwdBkwdPos,FrwdBkwdPosMax,FrwdBkwdPosMin,HdrstUpwdPos,HdrstUpwdPosMax,HdrstUpwdPosMin,LgrstUpwdPos,LgrstUpwdPosMax,LgrstUpwdPosMin,LtwdRtwdPos,LtwdRtwdPosMax,LtwdRtwdPosMin
  Bus Selector3 : BusSelector  OutputSignals=INTMSecRwRtSt
  Bus Selector4 : BusSelector  OutputSignals=BkReclnUpwdDnwdMovConfig,ArmTouchMovConfig,FrwdBkwdMovConfig,LgrstUpwdMovConfig,LtwdRtwdMovConfig
  Logical Operator3 : Logic  Operator=OR  AllPortsSameDT=off  OutDataTypeStr=boolean
  PA_KeSMSuMdMotFinshdTm_Val : Constant  Value=KeSMSuMdMotFinshdTm_Val
  PA_KeSMSuMdRetryTm1_Val : Constant  Value=KeSMSuMdRetryTm1_Val
  PA_KeSMSuModeReqDurgTm_Val : Constant  Value=KeSMSuModeReqDurgTm_Val
  PA_KeSMSuSecRwStArmTochPosDelta_Val : Constant  Value=KeSMSuSecRwStArmTochPosDelta_Val
  PA_KeSMSuSecRwStBackPosDelta_Val : Constant  Value=KeSMSuSecRwStBackPosDelta_Val
  PA_KeSMSuSecRwStFwdBkwdPosDelta_Val : Constant  Value=KeSMSuSecRwStFwdBkwdPosDelta_Val
  PA_KeSMSuSecRwStLegrestUpwdDwnwdPosDelta_Val : Constant  Value=KeSMSuSecRwStLegrestUpwdDwnwdPosDelta_Val
  PA_KeSMSuSecRwStLwdRwdPosDelta_Val : Constant  Value=KeSMSuSecRwStLwdRwdPosDelta_Val
  PA_KeSMSwDltTrgtPos_Val{1,3..5,17,19..22} (9 alike) : Constant  Value=KeSMSwPosInvalidVal_Val
  PA_KeSMSwDltTrgtPos_Val2 : Constant  Value=SeatChldLkSt.ChldLkSt_Unlock
  PA_KeSMSwDltTrgtPos_Val23 : Constant  OutDataTypeStr=boolean
  PA_KeSMSwDltTrgtPos_Val6 : Constant  Value=SeatChldLkSt.ChldLkSt_Unlock
  PA_KeSMSwDltTrgtPos_Val7 : Constant  Value=0  OutDataTypeStr=boolean
  PA_KeSMSwDltTrgtPos_Val8 : Constant  Value=0  OutDataTypeStr=boolean
  R2Rt_LtwdRtwd_Step2 : Lib/CommonUsed  SystemSampleTime=-1
  Terminator{,1..3,5} (5 alike) : Terminator
  Unit Delay : UnitDelay  SampleTime=-1
  R2RtSt_Step2_ini : Outport
  R2Rt_Step2_done : Outport  Port=2
  R2Rt_TrgtPoss : Outport  Port=3  VectorParamsAs1DForOutWhenUnconnected=on
  IfVeSMSbSecRwRtStRclCmdSrv_Val_writeRaw : Outport  Port=4
  wires:
  PA_KeSMSwDltTrgtPos_Val21/1 -> Bus Creator/4  "SecRwRtStCshnRrUpwdDnwdTrgtPos"
  PA_KeSMSwDltTrgtPos_Val20/1 -> Bus Creator/3  "SecRwRtStCshnFrntUpwdDnwdTrgtPos"
  PA_KeSMSwDltTrgtPos_Val1/1 -> Bus Creator/1  "SecRwRtStBkReclnUpwdDnwdTrgtPos"
  PA_KeSMSwDltTrgtPos_Val19/1 -> Bus Creator/2  "SecRwRtStBlstOtwdInwdTrgtPos"
  PA_KeSMSwDltTrgtPos_Val4/1 -> Bus Creator/7  "SecRwRtStLgrstUpwdDnwdTrgtPos"
  PA_KeSMSwDltTrgtPos_Val22/1 -> Bus Creator/6  "SecRwRtStHdrstUpwdDnwdTrgtPos"
  [R2Rt_LtwdRtwd_TarPos] -> Bus Creator/8  "SecRwRtStLtwdRtwdTrgtPos"
  PA_KeSMSwDltTrgtPos_Val3/1 -> Bus Creator/5  "SecRwRtStFrwdBkwdTrgtPos"
  Bus Creator/1 -> R2Rt_TrgtPoss/1
  R2Rt_LtwdRtwd_Step2/4 -> [Step2done_2]
  R2Rt_LtwdRtwd_Step2/2 -> Terminator5/1
  R2Rt_LtwdRtwd_Step2/1 -> [LtwdRtwd_inidone_Step2]
  R2Rt_LtwdRtwd_Step2/3 -> [R2Rt_LtwdRtwd_TarPos]
  [Tick] -> R2Rt_LtwdRtwd_Step2/11
  PA_KeSMSwDltTrgtPos_Val17/1 -> R2Rt_LtwdRtwd_Step2/10
  PA_KeSMSwDltTrgtPos_Val7/1 -> R2Rt_LtwdRtwd_Step2/9
  [KeSMSuSecRwStLwdRwdPosDelta_Val] -> R2Rt_LtwdRtwd_Step2/7
  [K_LtwdRtwdPos] -> R2Rt_LtwdRtwd_Step2/6
  [K_LtwdRtwdPosMax] -> R2Rt_LtwdRtwd_Step2/5
  [K_LtwdRtwdPosMin] -> R2Rt_LtwdRtwd_Step2/4
  [SecRwRtStLtwdRtwdPosV] -> R2Rt_LtwdRtwd_Step2/8
  [SecRwRtStLtwdRtwdPos] -> R2Rt_LtwdRtwd_Step2/3
  [Step1En] -> R2Rt_LtwdRtwd_Step2/2
  [Trig] -> R2Rt_LtwdRtwd_Step2/1
  Bus Selector/2 -> [SecRwRtStFrwdBkwdPos]  "<IfVeSMSuSecRwRtStFrwdBkwdPos_Val_read>"
  Bus Selector/3 -> [SecRwRtStHPassStUpwdDnwdPos]  "<IfVeSMSuSecRwRtStHPassStUpwdDnwdPos_Val_read>"
  Bus Selector1/5 -> [SecRwRtStLtwdRtwdPosV]  "<IfVeSMSuSecRwRtStLtwdRtwdPosV_Val_read>"
  SecRwRtStPoss/1 -> Bus Selector/1
  Bus Selector/5 -> [SecRwRtStLtwdRtwdPos]  "<IfVeSMSuSecRwRtStLtwdRtwdPos_Val_read>"
  Bus Selector1/4 -> [SecRwRtStLgrstUpwdDnwdPosV]  "<IfVeSMSuSecRwRtStLgrstUpwdDnwdPosV_Val_read>"
  Bus Selector/1 -> [SecRwRtStBkReclnUpwdDnwdPos]  "<IfVeSMSuSecRwRtStBkReclnUpwdDnwdPos_Val_read>"
  Bus Selector1/1 -> [SecRwRtStBkReclnUpwdDnwdPosV]  "<IfVeSMSuSecRwRtStBkReclnUpwdDnwdPosV_Val_read>"
  Bus Selector/4 -> [SecRwRtStLgrstUpwdDnwdPos]  "<IfVeSMSuSecRwRtStLgrstUpwdDnwdPos_Val_read>"
  Bus Selector1/3 -> [SecRwRtStHPassStUpwdDnwdPosV]  "<IfVeSMSuSecRwRtStHPassStUpwdDnwdPosV_Val_read>"
  SecRwRtStPossV/1 -> Bus Selector1/1
  Bus Selector1/2 -> [SecRwRtStFrwdBkwdPosV]  "<IfVeSMSuSecRwRtStFrwdBkwdPosV_Val_read>"
  Mode_Trig/1 -> [Trig]
  SecRwRtStChldLkRsp_L/1 -> Terminator/1
  PA_KeSMSwDltTrgtPos_Val2/1 -> Terminator1/1
  Step1En/1 -> [Step1En]
  PA_KeSMSwDltTrgtPos_Val23/1 -> IfVeSMSbSecRwRtStRclCmdSrv_Val_writeRaw/1
  PA_KeSMSuModeReqDurgTm_Val/1 -> [Tick]
  PA_KeSMSwDltTrgtPos_Val5/1 -> Bus Creator/9  "SecRwRtStArmScrnTrgtPos"
  PA_KeSMSuSecRwStBackPosDelta_Val/1 -> [KeSMSuSecRwStBackPosDelta_Val]
  PA_KeSMSuMdMotFinshdTm_Val/1 -> [KeSMSuMdMotFinshdTm_Val]
  PA_KeSMSuSecRwStFwdBkwdPosDelta_Val/1 -> [KeSMSuSecRwStFwdBkwdPosDelta_Val]
  PA_KeSMSuSecRwStLwdRwdPosDelta_Val/1 -> [KeSMSuSecRwStLwdRwdPosDelta_Val]
  PA_KeSMSuSecRwStArmTochPosDelta_Val/1 -> [KeSMSuSecRwStArmTochPosDelta_Val]
  PA_KeSMSuSecRwStLegrestUpwdDwnwdPosDelta_Val/1 -> [KeSMSuSecRwStLegrestUpwdDwnwdPosDelta_Val]
  [KeSMSuMdMotFinshdTm_Val] -> R2Rt_LtwdRtwd_Step2/12
  Bus Selector/6 -> [SecRwRtStArmScrnPos]  "<SecRwRtStArmScrnPos_Val_read>"
  Bus Selector1/6 -> [SecRwRtStArmScrnPosV]  "<SecRwRtStArmScrnPosV_Val_read>"
  Bus Selector2/1 -> [K_ArmScrnPos]  "<ArmScrnPos>"
  Bus Selector2/18 -> [K_LtwdRtwdPosMin]  "<LtwdRtwdPosMin>"
  Bus Selector2/16 -> [K_LtwdRtwdPos]  "<LtwdRtwdPos>"
  Bus Selector2/15 -> [K_LgrstUpwdPosMin]  "<LgrstUpwdPosMin>"
  Bus Selector2/17 -> [K_LtwdRtwdPosMax]  "<LtwdRtwdPosMax>"
  Bus Selector2/12 -> [K_HdrstUpwdPosMin]  "<HdrstUpwdPosMin>"
  Bus Selector2/13 -> [K_LgrstUpwdPos]  "<LgrstUpwdPos>"
  Bus Selector2/11 -> [K_HdrstUpwdPosMax]  "<HdrstUpwdPosMax>"
  Bus Selector2/14 -> [K_LgrstUpwdPosMax]  "<LgrstUpwdPosMax>"
  Bus Selector2/10 -> [K_HdrstUpwdPos]  "<HdrstUpwdPos>"
  Bus Selector2/4 -> [K_BkReclnUpwdDnwdPos]  "<BkReclnUpwdDnwdPos>"
  Bus Selector2/9 -> [K_FrwdBkwdPosMin]  "<FrwdBkwdPosMin>"
  Bus Selector2/5 -> [K_BkReclnUpwdDnwdPosMax]  "<BkReclnUpwdDnwdPosMax>"
  Bus Selector2/8 -> [K_FrwdBkwdPosMax]  "<FrwdBkwdPosMax>"
  Bus Selector3/1 -> Bus Selector2/1  "<INTMSecRwRtSt>"
  Bus Selector2/7 -> [K_FrwdBkwdPos]  "<FrwdBkwdPos>"
  Bus Selector2/3 -> [K_ArmScrnPosMin]  "<ArmScrnPosMin>"
  Bus Selector2/2 -> [K_ArmScrnPosMax]  "<ArmScrnPosMax>"
  Bus Selector2/6 -> [K_BkReclnUpwdDnwdPosMin]  "<BkReclnUpwdDnwdPosMin>"
  ModeStCalib_2R/1 -> Bus Selector3/1
  PA_KeSMSwDltTrgtPos_Val8/1 -> R2Rt_LtwdRtwd_Step2/13
  StConfig/1 -> Bus Selector4/1
  Bus Selector4/4 -> [LgrstUpwdMovConfig]  "<LgrstUpwdMovConfig>"
  Bus Selector4/3 -> [FrwdBkwdMovConfig]  "<FrwdBkwdMovConfig>"
  Bus Selector4/2 -> [ArmTouchMovConfig]  "<ArmTouchMovConfig>"
  Bus Selector4/1 -> [BkReclnUpwdDnwdMovConfig]  "<BkReclnUpwdDnwdMovConfig>"
  Bus Selector4/5 -> [LtwdRtwdMovConfig]  "<LtwdRtwdMovConfig>"
  [LtwdRtwdMovConfig] -> R2Rt_LtwdRtwd_Step2/14
  [Step2done_2] -> Unit Delay/1
  SecRwRtStChldLkRsp_R/1 -> Terminator2/1
  PA_KeSMSwDltTrgtPos_Val6/1 -> Terminator3/1
  [CntLow] -> R2Rt_LtwdRtwd_Step2/15
  PA_KeSMSuMdRetryTm1_Val/1 -> [CntLow]
  [LtwdRtwd_inidone_Step2] -> Logical Operator3/1, R2RtSt_Step2_ini/1
  Unit Delay/1 -> Logical Operator3/2
  Logical Operator3/1 -> R2Rt_Step2_done/1

== system ModeAdjust/ModeAdjustRunnable_sys/ModeAdjust/INTMR/R2Lt ==
  note: %1锁，2未锁
  Mode_Trig : Inport
  Step1En : Inport  Port=2
  SecRwLtStsPoss : Inport  Port=3
  SecRwLtStPossV : Inport  Port=4
  SecRwRtStChldLkRsp_L : Inport  Port=5
  ModeStCalib_2L : Inport  Port=6
  StConfig : Inport  Port=7
  SecRwRtStChldLkRsp_R : Inport  Port=8
  Bus Creator : BusCreator  Inputs=9  OutDataTypeStr=Bus: SecRwLfSeatPos
  Bus Selector : BusSelector  OutputSignals=IfVeSMSuSecRwLtStBkReclnUpwdDnwdPos_Val_read,IfVeSMSuSecRwLtStFrwdBkwdPos_Val_read,IfVeSMSuSecRwLtStHPassStUpwdDnwdPos_Val_read,IfVeSMSuSecRwLtStLgrstUpwdDnwdPos_Val_read,IfVeSMSuSecRwLtStLtwdRtwdPos_Val_read,IfVeSMSuSecRwLtStArmScrnPos_Val_read
  Bus Selector1 : BusSelector  OutputSignals=IfVeSMSuSecRwLtStBkReclnUpwdDnwdPosV_Val_read,IfVeSMSuSecRwLtStFrwdBkwdPosV_Val_read,IfVeSMSuSecRwLtStHPassStUpwdDnwdPosV_Val_read,IfVeSMSuSecRwLtStLgrstUpwdDnwdPosV_Val_read,IfVeSMSuSecRwLtStLtwdRtwdPosV_Val_read,IfVeSMSuSecRwLtStArmScrnPosV_Val_read
  Bus Selector2 : BusSelector  OutputSignals=ArmScrnPos,ArmScrnPosMax,ArmScrnPosMin,BkReclnUpwdDnwdPos,BkReclnUpwdDnwdPosMax,BkReclnUpwdDnwdPosMin,FrwdBkwdPos,FrwdBkwdPosMax,FrwdBkwdPosMin,HdrstUpwdPos,HdrstUpwdPosMax,HdrstUpwdPosMin,LgrstUpwdPos,LgrstUpwdPosMax,LgrstUpwdPosMin,LtwdRtwdPos,LtwdRtwdPosMax,LtwdRtwdPosMin
  Bus Selector3 : BusSelector  OutputSignals=INTMRSecRwLtSt
  Bus Selector4 : BusSelector  OutputSignals=BkReclnUpwdDnwdMovConfig,ArmTouchMovConfig,FrwdBkwdMovConfig,LgrstUpwdMovConfig,LtwdRtwdMovConfig
  Logical Operator3 : Logic  Operator=OR  AllPortsSameDT=off  OutDataTypeStr=boolean
  PA_KeSMSuMdMotFinshdTm_Val : Constant  Value=KeSMSuMdMotFinshdTm_Val
  PA_KeSMSuMdRetryTm1_Val : Constant  Value=KeSMSuMdRetryTm1_Val
  PA_KeSMSuModeReqDurgTm_Val : Constant  Value=KeSMSuModeReqDurgTm_Val
  PA_KeSMSuSecRwStArmTochPosDelta_Val : Constant  Value=KeSMSuSecRwStArmTochPosDelta_Val
  PA_KeSMSuSecRwStBackPosDelta_Val : Constant  Value=KeSMSuSecRwStBackPosDelta_Val
  PA_KeSMSuSecRwStFwdBkwdPosDelta_Val : Constant  Value=KeSMSuSecRwStFwdBkwdPosDelta_Val
  PA_KeSMSuSecRwStLegrestUpwdDwnwdPosDelta_Val : Constant  Value=KeSMSuSecRwStLegrestUpwdDwnwdPosDelta_Val
  PA_KeSMSuSecRwStLwdRwdPosDelta_Val : Constant  Value=KeSMSuSecRwStLwdRwdPosDelta_Val
  PA_KeSMSwDltTrgtPos_Val{1,3..4,6,14,18..21} (9 alike) : Constant  Value=KeSMSwPosInvalidVal_Val
  PA_KeSMSwDltTrgtPos_Val2 : Constant  Value=SeatChldLkSt.ChldLkSt_Unlock
  PA_KeSMSwDltTrgtPos_Val5 : Constant  OutDataTypeStr=boolean
  PA_KeSMSwDltTrgtPos_Val7 : Constant  Value=SeatChldLkSt.ChldLkSt_Unlock
  PA_KeSMSwDltTrgtPos_Val8 : Constant  Value=0  OutDataTypeStr=boolean
  PA_KeSMSwDltTrgtPos_Val9 : Constant  Value=0  OutDataTypeStr=boolean
  R2LtSt_LtwdRtwd_Step3 : Lib/CommonUsed  SystemSampleTime=-1
  Terminator{,1..4} (5 alike) : Terminator
  Unit Delay : UnitDelay  SampleTime=-1
  R2Lt_Ini : Outport
  R2Lt_Step2_done : Outport  Port=2
  R2Lt_TrgtPoss : Outport  Port=3  VectorParamsAs1DForOutWhenUnconnected=on
  IfVeSMSuSecRwLtStRclCmdSrv_Val_writeRaw : Outport  Port=4
  wires:
  Logical Operator3/1 -> R2Lt_Step2_done/1
  Unit Delay/1 -> Logical Operator3/2
  [LtwdRtwd_inidone] -> R2Lt_Ini/1, Logical Operator3/1
  PA_KeSMSuMdRetryTm1_Val/1 -> [CntLow]
  [CntLow] -> R2LtSt_LtwdRtwd_Step3/15
  PA_KeSMSwDltTrgtPos_Val7/1 -> Terminator3/1
  SecRwRtStChldLkRsp_R/1 -> Terminator2/1
  [LtwdRtwdMovConfig] -> R2LtSt_LtwdRtwd_Step3/14
  Bus Selector4/5 -> [LtwdRtwdMovConfig]  "<LtwdRtwdMovConfig>"
  Bus Selector4/1 -> [BkReclnUpwdDnwdMovConfig]  "<BkReclnUpwdDnwdMovConfig>"
  Bus Selector4/2 -> [ArmTouchMovConfig]  "<ArmTouchMovConfig>"
  Bus Selector4/3 -> [FrwdBkwdMovConfig]  "<FrwdBkwdMovConfig>"
  Bus Selector4/4 -> [LgrstUpwdMovConfig]  "<LgrstUpwdMovConfig>"
  StConfig/1 -> Bus Selector4/1
  PA_KeSMSwDltTrgtPos_Val9/1 -> R2LtSt_LtwdRtwd_Step3/13
  ModeStCalib_2L/1 -> Bus Selector3/1
  Bus Selector2/6 -> [K_BkReclnUpwdDnwdPosMin]  "<BkReclnUpwdDnwdPosMin>"
  Bus Selector2/2 -> [K_ArmScrnPosMax]  "<ArmScrnPosMax>"
  Bus Selector2/3 -> [K_ArmScrnPosMin]  "<ArmScrnPosMin>"
  Bus Selector2/7 -> [K_FrwdBkwdPos]  "<FrwdBkwdPos>"
  Bus Selector3/1 -> Bus Selector2/1  "<INTMRSecRwLtSt>"
  Bus Selector2/8 -> [K_FrwdBkwdPosMax]  "<FrwdBkwdPosMax>"
  Bus Selector2/5 -> [K_BkReclnUpwdDnwdPosMax]  "<BkReclnUpwdDnwdPosMax>"
  Bus Selector2/9 -> [K_FrwdBkwdPosMin]  "<FrwdBkwdPosMin>"
  Bus Selector2/4 -> [K_BkReclnUpwdDnwdPos]  "<BkReclnUpwdDnwdPos>"
  Bus Selector2/10 -> [K_HdrstUpwdPos]  "<HdrstUpwdPos>"
  Bus Selector2/14 -> [K_LgrstUpwdPosMax]  "<LgrstUpwdPosMax>"
  Bus Selector2/11 -> [K_HdrstUpwdPosMax]  "<HdrstUpwdPosMax>"
  Bus Selector2/13 -> [K_LgrstUpwdPos]  "<LgrstUpwdPos>"
  Bus Selector2/12 -> [K_HdrstUpwdPosMin]  "<HdrstUpwdPosMin>"
  Bus Selector2/17 -> [K_LtwdRtwdPosMax]  "<LtwdRtwdPosMax>"
  Bus Selector2/15 -> [K_LgrstUpwdPosMin]  "<LgrstUpwdPosMin>"
  Bus Selector2/16 -> [K_LtwdRtwdPos]  "<LtwdRtwdPos>"
  Bus Selector2/18 -> [K_LtwdRtwdPosMin]  "<LtwdRtwdPosMin>"
  Bus Selector2/1 -> [K_ArmScrnPos]  "<ArmScrnPos>"
  Bus Selector1/6 -> [SecRwLtStArmScrnPosV]  "<IfVeSMSuSecRwLtStArmScrnPosV_Val_read>"
  Bus Selector/6 -> [SecRwLtStArmScrnPos]  "<IfVeSMSuSecRwLtStArmScrnPos_Val_read>"
  [KeSMSuMdMotFinshdTm_Val] -> R2LtSt_LtwdRtwd_Step3/12
  PA_KeSMSuSecRwStLegrestUpwdDwnwdPosDelta_Val/1 -> [KeSMSuSecRwStLegrestUpwdDwnwdPosDelta_Val]
  PA_KeSMSuSecRwStArmTochPosDelta_Val/1 -> [KeSMSuSecRwStArmTochPosDelta_Val]
  PA_KeSMSuSecRwStLwdRwdPosDelta_Val/1 -> [KeSMSuSecRwStLwdRwdPosDelta_Val]
  PA_KeSMSuSecRwStFwdBkwdPosDelta_Val/1 -> [KeSMSuSecRwStFwdBkwdPosDelta_Val]
  PA_KeSMSuMdMotFinshdTm_Val/1 -> [KeSMSuMdMotFinshdTm_Val]
  PA_KeSMSuSecRwStBackPosDelta_Val/1 -> [KeSMSuSecRwStBackPosDelta_Val]
  PA_KeSMSwDltTrgtPos_Val6/1 -> Bus Creator/9  "SecRwLtStArmScrnTrgtPos"
  PA_KeSMSuModeReqDurgTm_Val/1 -> [Tick]
  PA_KeSMSwDltTrgtPos_Val5/1 -> IfVeSMSuSecRwLtStRclCmdSrv_Val_writeRaw/1
  Step1En/1 -> [Step1En]
  Mode_Trig/1 -> [Trig]
  Bus Selector1/3 -> [SecRwLtStHPassStUpwdDnwdPosV]  "<IfVeSMSuSecRwLtStHPassStUpwdDnwdPosV_Val_read>"
  Bus Selector/5 -> [SecRwLtStLtwdRtwdPos]  "<IfVeSMSuSecRwLtStLtwdRtwdPos_Val_read>"
  SecRwLtStsPoss/1 -> Bus Selector/1
  Bus Selector1/4 -> [SecRwLtStLgrstUpwdDnwdPosV]  "<IfVeSMSuSecRwLtStLgrstUpwdDnwdPosV_Val_read>"
  SecRwLtStPossV/1 -> Bus Selector1/1
  Bus Selector/3 -> [SecRwLtStHPassStUpwdDnwdPos]  "<IfVeSMSuSecRwLtStHPassStUpwdDnwdPos_Val_read>"
  Bus Selector1/5 -> [SecRwLtStLtwdRtwdPosV]  "<IfVeSMSuSecRwLtStLtwdRtwdPosV_Val_read>"
  Bus Selector/4 -> [SecRwLtStLgrstUpwdDnwdPos]  "<IfVeSMSuSecRwLtStLgrstUpwdDnwdPos_Val_read>"
  Bus Selector/2 -> [SecRwLtStFrwdBkwdPos]  "<IfVeSMSuSecRwLtStFrwdBkwdPos_Val_read>"
  Bus Selector1/1 -> [SecRwLtStBkReclnUpwdDnwdPosV]  "<IfVeSMSuSecRwLtStBkReclnUpwdDnwdPosV_Val_read>"
  Bus Selector1/2 -> [SecRwLtStFrwdBkwdPosV]  "<IfVeSMSuSecRwLtStFrwdBkwdPosV_Val_read>"
  Bus Selector/1 -> [SecRwLtStBkReclnUpwdDnwdPos]  "<IfVeSMSuSecRwLtStBkReclnUpwdDnwdPos_Val_read>"
  SecRwRtStChldLkRsp_L/1 -> Terminator/1
  PA_KeSMSwDltTrgtPos_Val2/1 -> Terminator1/1
  [K_LtwdRtwdPosMax] -> R2LtSt_LtwdRtwd_Step3/5
  [K_LtwdRtwdPos] -> R2LtSt_LtwdRtwd_Step3/6
  [K_LtwdRtwdPosMin] -> R2LtSt_LtwdRtwd_Step3/4
  [SecRwLtStLtwdRtwdPos] -> R2LtSt_LtwdRtwd_Step3/3
  [SecRwLtStLtwdRtwdPosV] -> R2LtSt_LtwdRtwd_Step3/8
  [Trig] -> R2LtSt_LtwdRtwd_Step3/1
  PA_KeSMSwDltTrgtPos_Val14/1 -> R2LtSt_LtwdRtwd_Step3/10
  [Tick] -> R2LtSt_LtwdRtwd_Step3/11
  [KeSMSuSecRwStLwdRwdPosDelta_Val] -> R2LtSt_LtwdRtwd_Step3/7
  PA_KeSMSwDltTrgtPos_Val8/1 -> R2LtSt_LtwdRtwd_Step3/9
  R2LtSt_LtwdRtwd_Step3/4 -> [LtwdRtwd_done]
  R2LtSt_LtwdRtwd_Step3/1 -> [LtwdRtwd_inidone]
  R2LtSt_LtwdRtwd_Step3/3 -> [R2LtSt_LtwdRtwd_TarPos]
  [Step1En] -> R2LtSt_LtwdRtwd_Step3/2
  [LtwdRtwd_done] -> Unit Delay/1
  R2LtSt_LtwdRtwd_Step3/2 -> Terminator4/1
  PA_KeSMSwDltTrgtPos_Val21/1 -> Bus Creator/6  "SecRwLtStHdrstUpwdDnwdTrgtPos"
  Bus Creator/1 -> R2Lt_TrgtPoss/1
  PA_KeSMSwDltTrgtPos_Val4/1 -> Bus Creator/7  "SecRwLtStLgrstUpwdDnwdTrgtPos"
  PA_KeSMSwDltTrgtPos_Val19/1 -> Bus Creator/3  "SecRwLtStCshnFrntUpwdDnwdTrgtPos"
  [R2LtSt_LtwdRtwd_TarPos] -> Bus Creator/8  "SecRwLtStLtwdRtwdTrgtPos"
  PA_KeSMSwDltTrgtPos_Val18/1 -> Bus Creator/2  "SecRwLtStBlstOtwdInwdTrgtPos"
  PA_KeSMSwDltTrgtPos_Val1/1 -> Bus Creator/1  "SecRwLtStBkReclnUpwdDnwdTrgtPos"
  PA_KeSMSwDltTrgtPos_Val3/1 -> Bus Creator/5  "SecRwLtStFrwdBkwdTrgtPos"
  PA_KeSMSwDltTrgtPos_Val20/1 -> Bus Creator/4  "SecRwLtStCshnRrUpwdDnwdTrgtPos"
